simulink model "regulator"  (R2021b)
settings: Solver=VariableStepAuto  StartTime=0.0  StopTime=8  RelTol=1e-3
values from neighbouring files (symbols this model uses):
  K = zeros(1, 3)    [stp01.m]
  start_x = [0 0 0]    [stp01.m]
  Tp = 0.5    [stp01.m]
undefined symbols (not defined in the file or in its folder): A_1, C_1
settings Model: Creator=USER  LastModifiedBy=USER

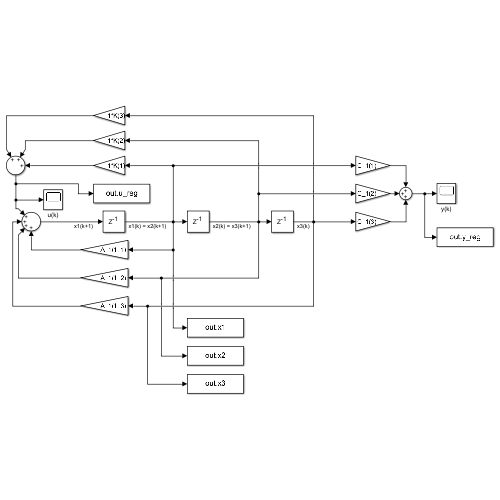
[thumbnail: Simulink's stored preview of the top-level diagram]
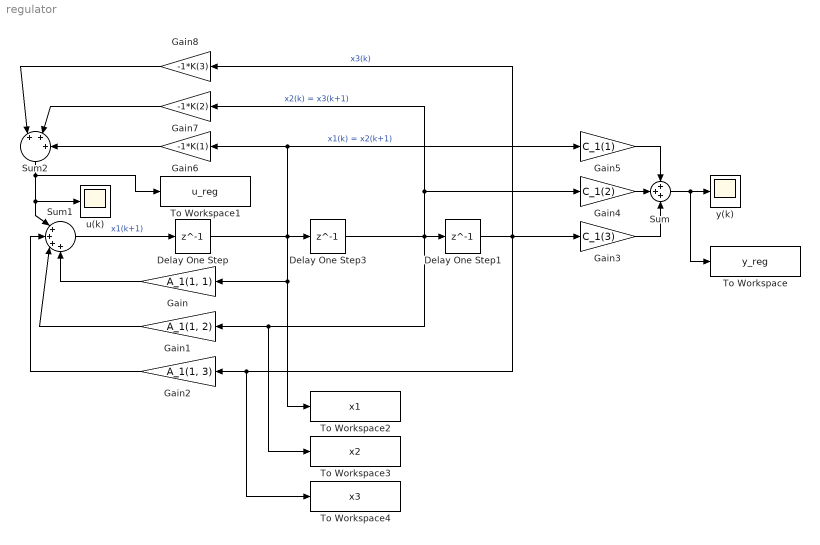
== system regulator ==
  Delay One Step : Delay  DelayLength=1  InitialCondition=start_x(1)  SampleTime=Tp
  Delay One Step1 : Delay  DelayLength=1  InitialCondition=start_x(3)  SampleTime=Tp
  Delay One Step3 : Delay  DelayLength=1  InitialCondition=start_x(2)  SampleTime=Tp
  Gain : Gain  Gain=A_1(1, 1)
  Gain1 : Gain  Gain=A_1(1, 2)
  Gain2 : Gain  Gain=A_1(1, 3)
  Gain3 : Gain  Gain=C_1(3)
  Gain4 : Gain  Gain=C_1(2)
  Gain5 : Gain  Gain=C_1(1)
  Gain6 : Gain  Gain=-1*K(1)
  Gain7 : Gain  Gain=-1*K(2)
  Gain8 : Gain  Gain=-1*K(3)
  Sum : Sum  Inputs=+++
  Sum1 : Sum  Inputs=|++++
  Sum2 : Sum  Inputs=|+++
  To Workspace : ToWorkspace  VariableName=y_reg  SaveFormat=Structure With Time  SampleTime=Tp
  To Workspace1 : ToWorkspace  VariableName=u_reg  SaveFormat=Structure With Time  SampleTime=Tp
  To Workspace2 : ToWorkspace  VariableName=x1  SaveFormat=Structure With Time  SampleTime=Tp
  To Workspace3 : ToWorkspace  VariableName=x2  SaveFormat=Structure With Time  SampleTime=Tp
  To Workspace4 : ToWorkspace  VariableName=x3  SaveFormat=Structure With Time  SampleTime=Tp
  u(k) : Scope
  y(k) : Scope
  wires:
  Sum/1 -> To Workspace/1, y(k)/1
  Gain/1 -> Sum1/4
  Gain4/1 -> Sum/2
  Delay One Step1/1 -> Gain8/1, Gain3/1, To Workspace4/1, Gain2/1  "x3(k)"
  Gain3/1 -> Sum/3
  Delay One Step3/1 -> Gain7/1, Gain4/1, To Workspace3/1, Gain1/1, Delay One Step1/1  "x2(k) = x3(k+1)"
  Gain5/1 -> Sum/1
  Delay One Step/1 -> Gain6/1, Gain5/1, To Workspace2/1, Gain/1, Delay One Step3/1  "x1(k) = x2(k+1)"
  Sum1/1 -> Delay One Step/1  "x1(k+1)"
  Gain1/1 -> Sum1/3
  Gain2/1 -> Sum1/2
  Sum2/1 -> To Workspace1/1, u(k)/1, Sum1/1
  Gain6/1 -> Sum2/3
  Gain7/1 -> Sum2/2
  Gain8/1 -> Sum2/1
